simulink model "slx15"  (R2023b)
settings: Solver=ode45  StartTime=0.0  StopTime=100  RelTol=1e-3
values from neighbouring files (symbols this model uses):
  Fx = 100    [m15.m]
  Fy = 0    [m15.m]
  l = length(u)    [m1.m]    (also in m15.m = 42)
  m = 0    [m14.m]    (also in m15.m = 1)
  x0 = [0; 0; l; 0;]    [m15.m]    (also in pendelSFunc.m = [])
settings Model: Creator=user  LastModifiedBy=user

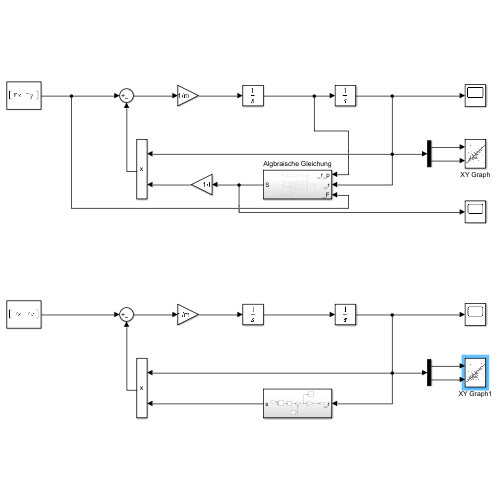
[thumbnail: Simulink's stored preview of the top-level diagram]
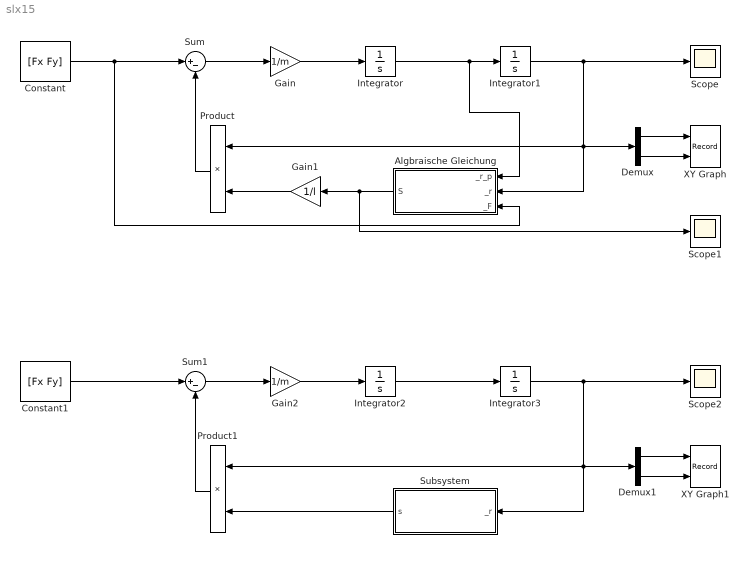
== system slx15 ==
  Algbraische Gleichung : Subsystem
  Constant : Constant  Value=[Fx Fy]
  Constant1 : Constant  Value=[Fx Fy]
  Demux : Demux  Outputs=2
  Demux1 : Demux  Outputs=2
  Gain : Gain  Gain=1/m
  Gain1 : Gain  Gain=1/l
  Gain2 : Gain  Gain=1/m
  Integrator : Integrator
  Integrator1 : Integrator  InitialCondition=x0([1,3])
  Integrator2 : Integrator
  Integrator3 : Integrator  InitialCondition=x0([1,3])
  Product : Product
  Product1 : Product
  Scope : Scope
  Scope1 : Scope
  Scope2 : Scope
  Subsystem : Subsystem
  Sum : Sum  Inputs=|+-
  Sum1 : Sum  Inputs=|+-
  XY Graph : Record  FileSettingsInternal="{\"entries\":[{\"content\":{\"excelSettings\":{\"content\":{},\"type\":\"Streamout.ExcelSettings\"}},\"type\":\"Streamout.FileSettingStorage\",\"uuid\":\"\"}],\"packageUris\":[\"http:\\/\\/schema.mathworks.com\\/mf0\\/streamout_blocks\\/R2020a\"],\"version\":\"1.0\"}"  Layout=[1 1]  SignalsInternal="{\"entries\":[{\"content\":{\"signals\":[{\"content\":{\"blockPath\":[],\"dimensions\":[1],\"domain\":\"\",\"lineColor\":\"#64d413\",\"port\":1,\"sid\":[\"\"],\"signalID\":4419,\"signalName\":\"Demux:1\"},\"type\":\"RecordBlkView.Signal\",\"uuid\":\"\"},{\"content\":{\"blockPath\":[],\"dimensions\":[1],\"domain\":\"\",\"lineColor\":\"#ff13a6\",\"port\":2,\"sid\":[\"\"],\"signalID\":4423,\"signalName\":\"Demux:2\"},\"type\":\"RecordBlkView.Signal\",\"uuid\":\"\"}]},\"type\":\"RecordBlkView.InputSignals\",\"uuid\":\"\"}],\"packageUris\":[\"http:\\/\\/schema.mathworks.com\\/mf0\\/streamout_blocks\\/R2020a\"],\"version\":\"1.0\"}"  VisualizationBindings="{\"xyplotplugin\":{\"info\":[{\"series\":[],\"subplotID\":1}]}}"  CompatibilityTag=XY
  XY Graph1 : Record  FileSettingsInternal="{\"entries\":[{\"content\":{\"excelSettings\":{\"content\":{},\"type\":\"Streamout.ExcelSettings\"}},\"type\":\"Streamout.FileSettingStorage\",\"uuid\":\"\"}],\"packageUris\":[\"http:\\/\\/schema.mathworks.com\\/mf0\\/streamout_blocks\\/R2020a\"],\"version\":\"1.0\"}"  Layout=[1 1]  SignalsInternal="{\"entries\":[{\"content\":{\"signals\":[{\"content\":{\"blockPath\":[],\"dimensions\":[1],\"domain\":\"\",\"lineColor\":\"#fe330a\",\"port\":1,\"sid\":[\"\"],\"signalID\":4427,\"signalName\":\"Demux1:1\"},\"type\":\"RecordBlkView.Signal\",\"uuid\":\"\"},{\"content\":{\"blockPath\":[],\"dimensions\":[1],\"domain\":\"\",\"lineColor\":\"#22b573\",\"port\":2,\"sid\":[\"\"],\"signalID\":4431,\"signalName\":\"Demux1:2\"},\"type\":\"RecordBlkView.Signal\",\"uuid\":\"\"}]},\"type\":\"RecordBlkView.InputSignals\",\"uuid\":\"\"}],\"packageUris\":[\"http:\\/\\/schema.mathworks.com\\/mf0\\/streamout_blocks\\/R2020a\"],\"version\":\"1.0\"}"  VisualizationBindings="{\"xyplotplugin\":{\"info\":[{\"series\":[],\"subplotID\":1}]}}"  CompatibilityTag=XY
  wires:
  Constant/1 -> Algbraische Gleichung/3(_F), Sum/1
  Sum/1 -> Gain/1
  Gain/1 -> Integrator/1
  Integrator/1 -> Algbraische Gleichung/1(_r_p), Integrator1/1
  Product/1 -> Sum/2
  Algbraische Gleichung/1(S) -> Scope1/1, Gain1/1
  Gain1/1 -> Product/2
  Demux/1 -> XY Graph/1
  Demux/2 -> XY Graph/2
  Integrator1/1 -> Demux/1, Product/1, Algbraische Gleichung/2(_r), Scope/1
  Integrator3/1 -> Scope2/1, Subsystem/1(_r), Product1/1, Demux1/1
  Demux1/2 -> XY Graph1/2
  Demux1/1 -> XY Graph1/1
  Subsystem/1(s) -> Product1/2
  Product1/1 -> Sum1/2
  Integrator2/1 -> Integrator3/1
  Gain2/1 -> Integrator2/1
  Sum1/1 -> Gain2/1
  Constant1/1 -> Sum1/1

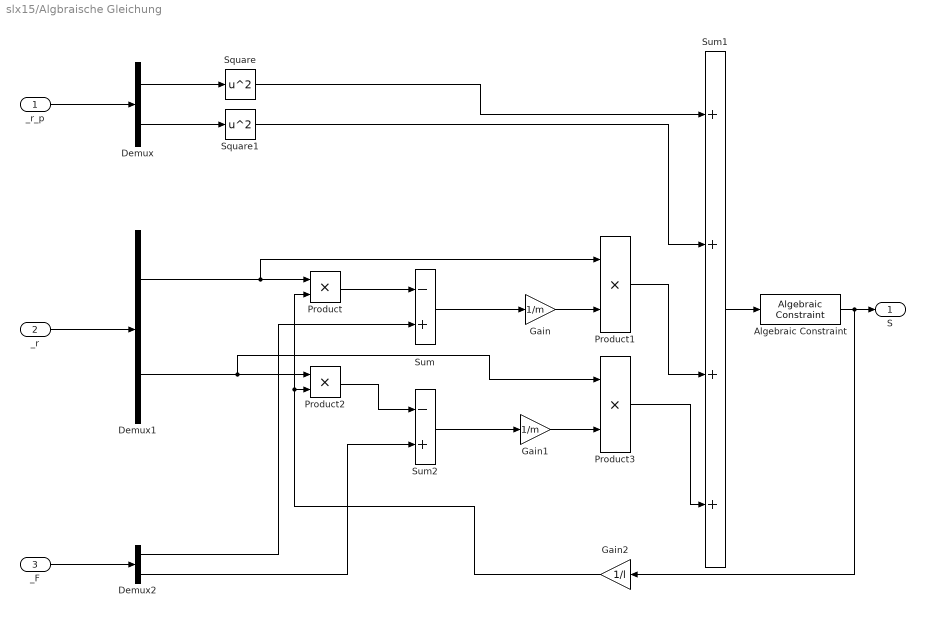
== system slx15/Algbraische Gleichung ==
  _r_p : Inport
  _r : Inport  Port=2
  _F : Inport  Port=3
  Algebraic Constraint : AlgebraicConstraint
  Demux : Demux  Outputs=2
  Demux1 : Demux  Outputs=2
  Demux2 : Demux  Outputs=2
  Gain : Gain  Gain=1/m
  Gain1 : Gain  Gain=1/m
  Gain2 : Gain  Gain=1/l
  Product{,1..3} (4 alike) : Product
  Square : Math  Operator=square
  Square1 : Math  Operator=square
  Sum : Sum  Inputs=-+
  Sum1 : Sum  Inputs=++++
  Sum2 : Sum  Inputs=-+
  S : Outport
  wires:
  _r_p/1 -> Demux/1
  _r/1 -> Demux1/1
  _F/1 -> Demux2/1
  Demux/1 -> Square/1
  Demux/2 -> Square1/1
  Demux1/1 -> Product1/1, Product/1
  Gain/1 -> Product1/2
  Product/1 -> Sum/1
  Sum/1 -> Gain/1
  Demux2/1 -> Sum/2
  Product1/1 -> Sum1/3
  Square/1 -> Sum1/1
  Square1/1 -> Sum1/2
  Demux1/2 -> Product3/1, Product2/1
  Product2/1 -> Sum2/1
  Demux2/2 -> Sum2/2
  Sum2/1 -> Gain1/1
  Gain1/1 -> Product3/2
  Product3/1 -> Sum1/4
  Algebraic Constraint/1 -> Gain2/1, S/1
  Sum1/1 -> Algebraic Constraint/1
  Gain2/1 -> Product2/2, Product/2

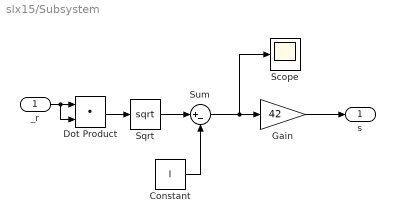
== system slx15/Subsystem ==
  _r : Inport
  Constant : Constant  Value=l
  Dot Product : DotProduct  OutDataTypeStr=Inherit: Inherit via internal rule
  Gain : Gain  Gain=42
  Scope : Scope
  Sqrt : Sqrt
  Sum : Sum  Inputs=|+-
  s : Outport
  wires:
  Gain/1 -> s/1
  _r/1 -> Dot Product/2, Dot Product/1
  Dot Product/1 -> Sqrt/1
  Sqrt/1 -> Sum/1
  Constant/1 -> Sum/2
  Sum/1 -> Scope/1, Gain/1
